simulink model "boucle_ouverte"  (R2018b)
settings: Solver=VariableStepAuto  StartTime=0.0  StopTime=10.0  RelTol=1e-3
values from neighbouring files (symbols this model uses):
  epsilon = 0.1    [parametres_tp2.m]
  omega = 0.02    [parametres_tp2.m]
settings Model: Creator=12003927  LastModifiedBy=12003927

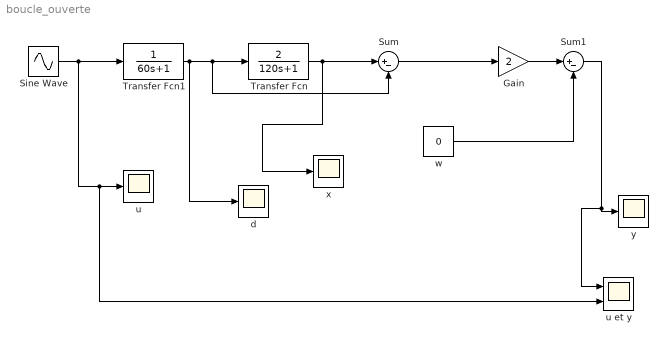
== system boucle_ouverte ==
  Gain : Gain  Gain=2
  Sine Wave : Sin  Amplitude=epsilon  Frequency=omega  SampleTime=0
  Sum : Sum  Inputs=|+-
  Sum1 : Sum  Inputs=|+-
  Transfer Fcn : TransferFcn  Numerator=2  Denominator=[120 1]
  Transfer Fcn1 : TransferFcn  Denominator=[60 1]
  d : Scope
  u : Scope
  u et y : Scope  NumInputPorts=2
  w : Constant  Value=0
  x : Scope
  y : Scope
  wires:
  Transfer Fcn1/1 -> d/1, Sum/2, Transfer Fcn/1
  Transfer Fcn/1 -> x/1, Sum/1
  Sum/1 -> Gain/1
  Gain/1 -> Sum1/1
  Sine Wave/1 -> u et y/2, u/1, Transfer Fcn1/1
  w/1 -> Sum1/2
  Sum1/1 -> u et y/1, y/1
